simulink model "ROS2ValetControllerExample"  (R2022b)
settings: Solver=FixedStepAuto  StartTime=0.0  StopTime=inf  RelTol=1e-3
model workspace (MAT data in the model file):
  SL_ROS_VariableLengthArrays_MaxSizes.CommonInfo.ArrayTruncateAction = 'EmitWarning'
  SL_ROS_VariableLengthArrays_MaxSizes.MsgTypeMap = containers.Map
  SL_ROS_VariableLengthArrays_MaxSizes.MsgTypeMap.serialization.keys = {'std_msgs/Float64MultiArray'}
  SL_ROS_VariableLengthArrays_MaxSizes.MsgTypeMap.serialization.values{1}.PropertyName = 'data'
  SL_ROS_VariableLengthArrays_MaxSizes.MsgTypeMap.serialization.values{1}.DataType = 'double'
  SL_ROS_VariableLengthArrays_MaxSizes.MsgTypeMap.serialization.values{1}.MaxLength = 1500
  SL_ROS_VariableLengthArrays_MaxSizes.MsgTypeMap.serialization.uniformity = 0
  SL_ROS_VariableLengthArrays_MaxSizes.MsgTypeMap.serialization.keyType = 'char'
  SL_ROS_VariableLengthArrays_MaxSizes.MsgTypeMap.serialization.valueType = 'any'
values from neighbouring files (symbols this model uses):
  directions = obj.DirectionsInternal    [ExampleHelperROSValetPathAnalyzer.m]
libraries: ros2lib x19, drivingvehiclecontroller x2
settings Model: PacingRate=1000  Creator=The MathWorks, Inc.  LastModifiedBy=The MathWorks, Inc.
settings SolverCC: AlgebraicLoopSolver=TrustRegion
settings OptimizationCC: EnhancedBackFolding=on  PassReuseOutputArgsAs=Individual arguments  ZeroExternalMemoryAtStartup=off  ZeroInternalMemoryAtStartup=off  MaxStackSize=64  OptimizeBlockOrder=speed  DifferentSizesBufferReuse=on  OptimizationCustomize=off  EfficientTunableParamExpr=on
settings DebuggingCC: ParameterTunabilityLossMsg=error  UnconnectedInputMsg=warning  UnconnectedOutputMsg=warning  UnconnectedLineMsg=warning  SFMachineParentedDataDiag=warning
settings ModelReferenceCC: EnableRefExpFcnMdlSchedulingChecks=on
settings SFSimCC: SimTargetLang=C++
settings RTWCC: Description=Embedded Coder  SystemTargetFile=ert.tlc  HardwareBoard=Robot Operating System 2 (ROS 2)  TLCOptions=-aInlineSetEventsForThisBaseRateFcn=TLC_FALSE -aSuppressMultiTaskScheduler=TLC_FALSE -aRateBasedStepFcn=1  TemplateMakefile=ert_default_tmf  GenerateReport=on  Toolchain=Colcon Tools  IncludeHyperlinkInReport=on  LaunchReport=on  TargetLang=C++  GenerateTraceInfo=on  GenerateTraceReport=on  GenerateTraceReportSl=on  GenerateTraceReportSf=on  GenerateTraceReportEml=on
settings CodeAppCC: ForceParamTrailComments=on  IgnoreCustomStorageClasses=off  OperatorAnnotations=on  SimulinkDataObjDesc=on  SFDataObjDesc=on  InsertBlockDesc=on
settings ERTTargetCC: CodeInterfacePackaging=C++ class  RootIOFormat=Structure reference

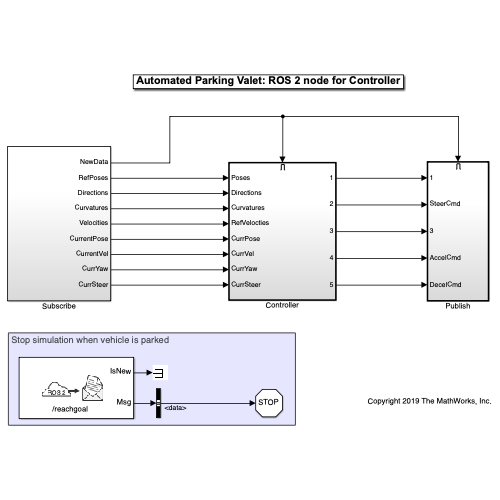
[thumbnail: Simulink's stored preview of the top-level diagram]
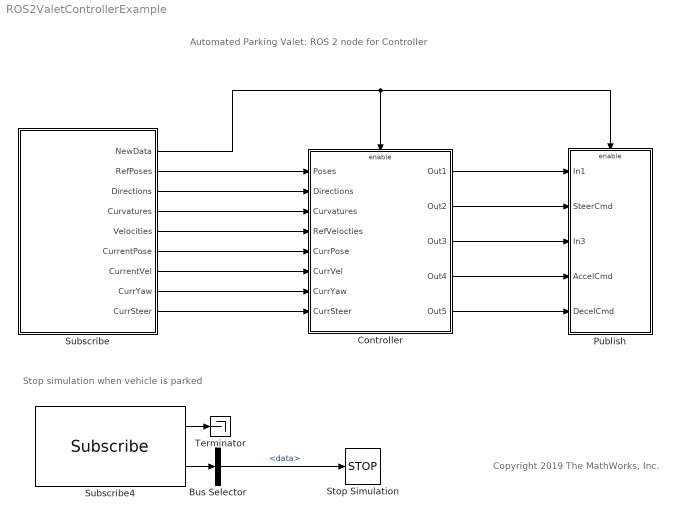
== system ROS2ValetControllerExample ==
  note: Copyright 2019 The MathWorks, Inc.
  note: Automated Parking Valet: ROS 2 node for Controller
  note: Stop simulation when vehicle is parked
  Bus Selector : BusSelector  OutputSignals=data
  Controller : Subsystem
  Publish : Subsystem
  Stop Simulation : Stop
  Subscribe : Subsystem
  Subscribe4 : ros2lib/Subscribe  topicSource=Specify your own  topic=/reachgoal  messageType=std_msgs/Bool  sampleTime=-1  QOSHistory=Keep last  QOSDepth=1  QOSReliability=Reliable  QOSDurability=Volatile
  Terminator : Terminator
  wires:
  Subscribe/1(NewData) -> Controller/Enable, Publish/Enable
  Subscribe/2(RefPoses) -> Controller/1(Poses)
  Subscribe/3(Directions) -> Controller/2(Directions)
  Subscribe/4(Curvatures) -> Controller/3(Curvatures)
  Subscribe/5(Velocities) -> Controller/4(RefVelocties)
  Subscribe/6(CurrentPose) -> Controller/5(CurrPose)
  Subscribe/7(CurrentVel) -> Controller/6(CurrVel)
  Subscribe/8(CurrYaw) -> Controller/7(CurrYaw)
  Subscribe/9(CurrSteer) -> Controller/8(CurrSteer)
  Subscribe4/2 -> Bus Selector/1
  Subscribe4/1 -> Terminator/1
  Bus Selector/1 -> Stop Simulation/1  "<data>"
  Controller/4(Out4) -> Publish/4(AccelCmd)
  Controller/5(Out5) -> Publish/5(DecelCmd)
  Controller/3(Out3) -> Publish/3(In3)
  Controller/2(Out2) -> Publish/2(SteerCmd)
  Controller/1(Out1) -> Publish/1(In1)

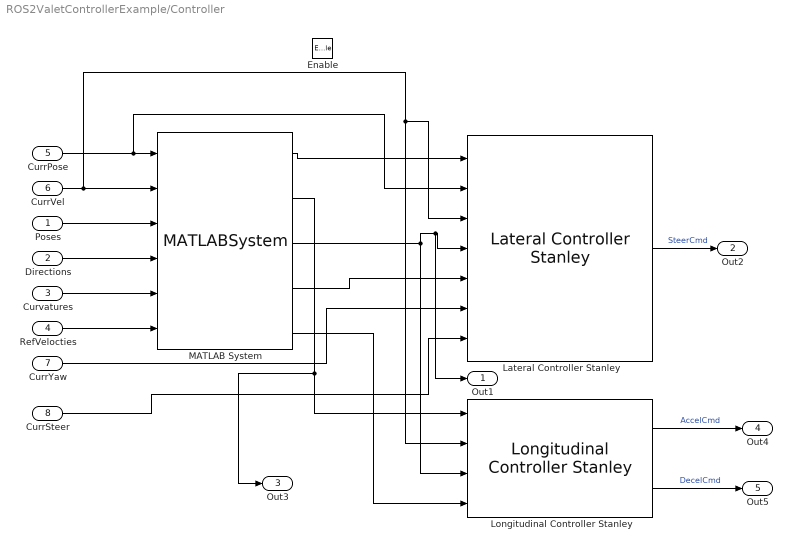
== system ROS2ValetControllerExample/Controller ==
  Poses : Inport
  Directions : Inport  Port=2
  Curvatures : Inport  Port=3
  RefVelocties : Inport  Port=4
  CurrPose : Inport  Port=5
  CurrVel : Inport  Port=6
  CurrYaw : Inport  Port=7
  CurrSteer : Inport  Port=8
  Enable : EnablePort
  Lateral Controller Stanley : drivingvehiclecontroller/Lateral Controller Stanley  ModelType=Dynamic bicycle model  PositionGainF=2  PositionGainR=2.5  YawRateGain=0.25  DelayGain=0.2  VehicleMass=1575  Lf=1.2  Lr=1.6  TireStiffness=19e3  Wheelbase=2.8  MaxSteeringAngle=35
  Longitudinal Controller Stanley : drivingvehiclecontroller/Longitudinal Controller Stanley  Kp=2.5  Ki=1  SampleTime=0.05  MaxAcceleration=3  MaxDeceleration=6
  MATLAB System : MATLABSystem  System=ExampleHelperROSValetPathAnalyzer  Wheelbase=2.8  HasResetOutput=on  SimulateUsing=Interpreted execution
      mask Type: ExampleHelperROSValetPathAnalyzer
      mask Display:
      | disp(['Helper' char(10) 'Path' char(10) 'Analyzer']);
      | port_label('input',1,'CurrPose');
      | port_label('input',2,'CurrVelocity');
      | port_label('input',3,'RefPoses');
      | port_label('input',4,'Directions');
      | port_label('input',5,'Curvatures');
      | port_label('input',6,'RefVelocities');
      | port_label('output',1,'RefPose');
      | port_label('output',2,'RefVelocity');
      | port_label('output',3,'Direction');
      | port_label('output',4,'Curvature');
      | port_label('output',5,'Reset');
  Out1 : Outport
  Out2 : Outport  Port=2
  Out3 : Outport  Port=3
  Out4 : Outport  Port=4
  Out5 : Outport  Port=5
  wires:
  MATLAB System/2 -> Longitudinal Controller Stanley/1, Out3/1
  MATLAB System/4 -> Lateral Controller Stanley/5
  MATLAB System/1 -> Lateral Controller Stanley/1
  MATLAB System/5 -> Longitudinal Controller Stanley/4
  Poses/1 -> MATLAB System/3
  CurrVel/1 -> Lateral Controller Stanley/3, Longitudinal Controller Stanley/2, MATLAB System/2
  CurrYaw/1 -> Lateral Controller Stanley/6
  CurrSteer/1 -> Lateral Controller Stanley/7
  CurrPose/1 -> Lateral Controller Stanley/2, MATLAB System/1
  Directions/1 -> MATLAB System/4
  Curvatures/1 -> MATLAB System/5
  RefVelocties/1 -> MATLAB System/6
  MATLAB System/3 -> Out1/1, Lateral Controller Stanley/4, Longitudinal Controller Stanley/3
  Lateral Controller Stanley/1 -> Out2/1  "SteerCmd"
  Longitudinal Controller Stanley/1 -> Out4/1  "AccelCmd"
  Longitudinal Controller Stanley/2 -> Out5/1  "DecelCmd"

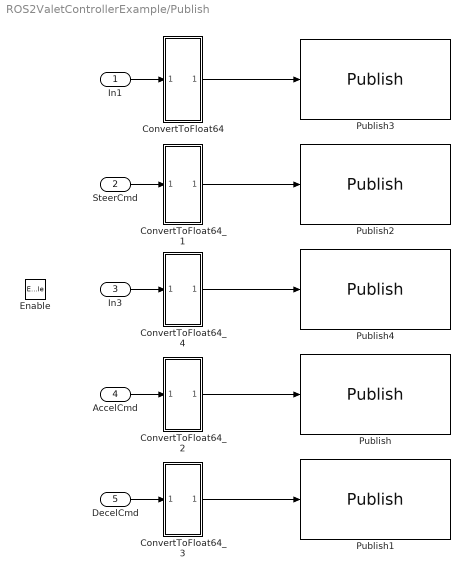
== system ROS2ValetControllerExample/Publish ==
  In1 : Inport
  SteerCmd : Inport  Port=2
  In3 : Inport  Port=3
  AccelCmd : Inport  Port=4
  DecelCmd : Inport  Port=5
  Enable : EnablePort
  ConvertToFloat64 : Subsystem
  ConvertToFloat64_1 : Subsystem
  ConvertToFloat64_2 : Subsystem
  ConvertToFloat64_3 : Subsystem
  ConvertToFloat64_4 : Subsystem
  Publish : ros2lib/Publish  topicSource=Specify your own  topic=/accelcmd  messageType=std_msgs/Float64  QOSHistory=Keep last  QOSDepth=1  QOSReliability=Reliable  QOSDurability=Volatile
  Publish1 : ros2lib/Publish  topicSource=Specify your own  topic=/decelcmd  messageType=std_msgs/Float64  QOSHistory=Keep last  QOSDepth=1  QOSReliability=Reliable  QOSDurability=Volatile
  Publish2 : ros2lib/Publish  topicSource=Specify your own  topic=/steeringangle  messageType=std_msgs/Float64  QOSHistory=Keep last  QOSDepth=1  QOSReliability=Reliable  QOSDurability=Volatile
  Publish3 : ros2lib/Publish  topicSource=Specify your own  topic=/vehdir  messageType=std_msgs/Float64  QOSHistory=Keep last  QOSDepth=1  QOSReliability=Reliable  QOSDurability=Volatile
  Publish4 : ros2lib/Publish  topicSource=Specify your own  topic=/refvelocity  messageType=std_msgs/Float64  QOSHistory=Keep last  QOSDepth=1  QOSReliability=Reliable  QOSDurability=Volatile
  wires:
  AccelCmd/1 -> ConvertToFloat64_2/1(In1)
  SteerCmd/1 -> ConvertToFloat64_1/1(In1)
  DecelCmd/1 -> ConvertToFloat64_3/1(In1)
  ConvertToFloat64_2/1(Out1) -> Publish/1
  ConvertToFloat64_4/1(Out1) -> Publish4/1
  ConvertToFloat64_1/1(Out1) -> Publish2/1
  ConvertToFloat64/1(Out1) -> Publish3/1
  In3/1 -> ConvertToFloat64_4/1(In1)
  ConvertToFloat64_3/1(Out1) -> Publish1/1
  In1/1 -> ConvertToFloat64/1(In1)

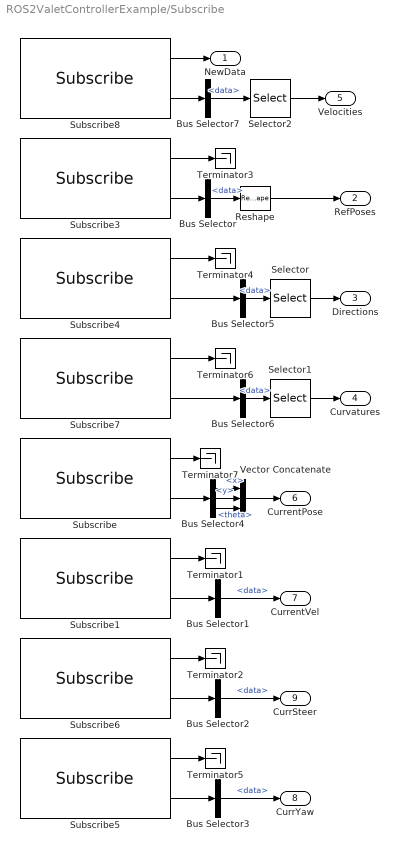
== system ROS2ValetControllerExample/Subscribe ==
  Bus Selector{,1..3,5..7} (7 alike) : BusSelector  OutputSignals=data
  Bus Selector4 : BusSelector  OutputSignals=x,y,theta
  Reshape : Reshape  OutputDimensionality=Customize  OutputDimensions=[500,3]
  Selector : Selector  InputPortWidth=1500  IndexOptions=Starting index (dialog)  Indices=1  OutputSizes=500
  Selector1 : Selector  InputPortWidth=1500  IndexOptions=Starting index (dialog)  Indices=1  OutputSizes=500
  Selector2 : Selector  InputPortWidth=1500  IndexOptions=Starting index (dialog)  Indices=1  OutputSizes=500
  Subscribe : ros2lib/Subscribe  topicSource=Select from ROS network  topic=/currentpose  messageType=geometry_msgs/Pose2D  sampleTime=-1  QOSHistory=Keep last  QOSDepth=1  QOSReliability=Reliable  QOSDurability=Volatile
  Subscribe1 : ros2lib/Subscribe  topicSource=Select from ROS network  topic=/currentvel  messageType=std_msgs/Float64  sampleTime=-1  QOSHistory=Keep last  QOSDepth=1  QOSReliability=Reliable  QOSDurability=Volatile
  Subscribe3 : ros2lib/Subscribe  topicSource=Specify your own  topic=/smoothpath  messageType=std_msgs/Float64MultiArray  sampleTime=-1  QOSHistory=Keep last  QOSDepth=1  QOSReliability=Reliable  QOSDurability=Volatile
  Subscribe4 : ros2lib/Subscribe  topicSource=Specify your own  topic=/directions  messageType=std_msgs/Float64MultiArray  sampleTime=-1  QOSHistory=Keep last  QOSDepth=1  QOSReliability=Reliable  QOSDurability=Volatile
  Subscribe5 : ros2lib/Subscribe  topicSource=Specify your own  topic=/curryawrate  messageType=std_msgs/Float64  sampleTime=-1  QOSHistory=Keep last  QOSDepth=1  QOSReliability=Reliable  QOSDurability=Volatile
  Subscribe6 : ros2lib/Subscribe  topicSource=Specify your own  topic=/currentsteering  messageType=std_msgs/Float64  sampleTime=-1  QOSHistory=Keep last  QOSDepth=1  QOSReliability=Reliable  QOSDurability=Volatile
  Subscribe7 : ros2lib/Subscribe  topicSource=Specify your own  topic=/curvatures  messageType=std_msgs/Float64MultiArray  sampleTime=-1  QOSHistory=Keep last  QOSDepth=1  QOSReliability=Reliable  QOSDurability=Volatile
  Subscribe8 : ros2lib/Subscribe  topicSource=Specify your own  topic=/velprofile  messageType=std_msgs/Float64MultiArray  sampleTime=-1  QOSHistory=Keep last  QOSDepth=1  QOSReliability=Reliable  QOSDurability=Volatile
  Terminator{1..7} (7 alike) : Terminator
  Vector Concatenate : Concatenate  NumInputs=3  Mode=Multidimensional array  ConcatenateDimension=2
  NewData : Outport  VectorParamsAs1DForOutWhenUnconnected=off
  RefPoses : Outport  Port=2  VectorParamsAs1DForOutWhenUnconnected=off
  Directions : Outport  Port=3  VectorParamsAs1DForOutWhenUnconnected=off
  Curvatures : Outport  Port=4  VectorParamsAs1DForOutWhenUnconnected=off
  Velocities : Outport  Port=5  VectorParamsAs1DForOutWhenUnconnected=off
  CurrentPose : Outport  Port=6  VectorParamsAs1DForOutWhenUnconnected=off
  CurrentVel : Outport  Port=7  VectorParamsAs1DForOutWhenUnconnected=off
  CurrYaw : Outport  Port=8  VectorParamsAs1DForOutWhenUnconnected=off
  CurrSteer : Outport  Port=9  VectorParamsAs1DForOutWhenUnconnected=off
  wires:
  Subscribe/1 -> Terminator7/1
  Subscribe1/2 -> Bus Selector1/1
  Subscribe1/1 -> Terminator1/1
  Subscribe3/1 -> Terminator3/1
  Subscribe4/1 -> Terminator4/1
  Subscribe5/1 -> Terminator5/1
  Subscribe5/2 -> Bus Selector3/1
  Subscribe6/2 -> Bus Selector2/1
  Subscribe6/1 -> Terminator2/1
  Subscribe7/1 -> Terminator6/1
  Subscribe8/1 -> NewData/1
  Bus Selector6/1 -> Selector1/1  "<data>"
  Bus Selector7/1 -> Selector2/1  "<data>"
  Bus Selector4/2 -> Vector Concatenate/2  "<y>"
  Bus Selector4/3 -> Vector Concatenate/3  "<theta>"
  Bus Selector4/1 -> Vector Concatenate/1  "<x>"
  Bus Selector5/1 -> Selector/1  "<data>"
  Subscribe/2 -> Bus Selector4/1
  Vector Concatenate/1 -> CurrentPose/1
  Bus Selector1/1 -> CurrentVel/1  "<data>"
  Bus Selector2/1 -> CurrSteer/1  "<data>"
  Bus Selector3/1 -> CurrYaw/1  "<data>"
  Bus Selector/1 -> Reshape/1  "<data>"
  Subscribe3/2 -> Bus Selector/1
  Reshape/1 -> RefPoses/1
  Subscribe4/2 -> Bus Selector5/1
  Selector/1 -> Directions/1
  Subscribe7/2 -> Bus Selector6/1
  Selector1/1 -> Curvatures/1
  Subscribe8/2 -> Bus Selector7/1
  Selector2/1 -> Velocities/1

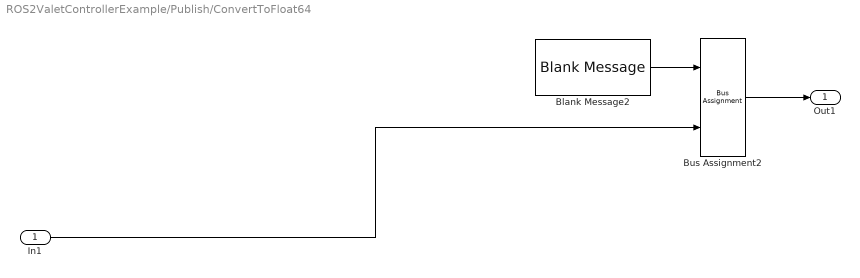
== system ROS2ValetControllerExample/Publish/ConvertToFloat64 ==
  In1 : Inport
  Blank Message2 : ros2lib/Blank Message  messageClass=Message  entityType=std_msgs/Float64  messageType=std_msgs/Float64  SampleTime=-1
  Bus Assignment2 : BusAssignment  AssignedSignals=data
  Out1 : Outport
  wires:
  Blank Message2/1 -> Bus Assignment2/1
  Bus Assignment2/1 -> Out1/1
  In1/1 -> Bus Assignment2/2

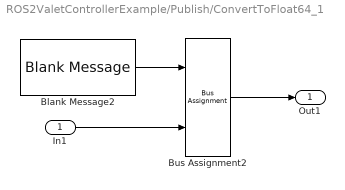
== system ROS2ValetControllerExample/Publish/ConvertToFloat64_1 ==
  In1 : Inport
  Blank Message2 : ros2lib/Blank Message  messageClass=Message  entityType=std_msgs/Float64  messageType=std_msgs/Float64  SampleTime=-1
  Bus Assignment2 : BusAssignment  AssignedSignals=data
  Out1 : Outport
  wires:
  In1/1 -> Bus Assignment2/2
  Bus Assignment2/1 -> Out1/1
  Blank Message2/1 -> Bus Assignment2/1

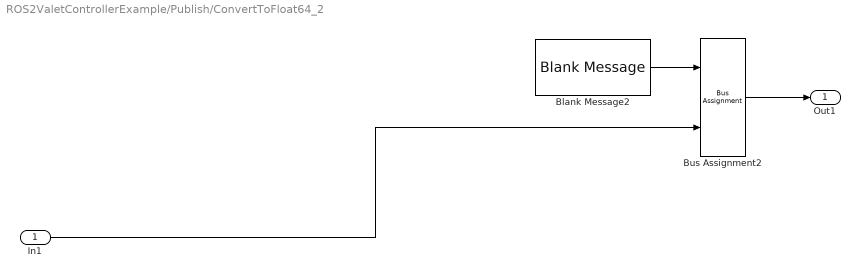
== system ROS2ValetControllerExample/Publish/ConvertToFloat64_2 ==
  In1 : Inport
  Blank Message2 : ros2lib/Blank Message  messageClass=Message  entityType=std_msgs/Float64  messageType=std_msgs/Float64  SampleTime=-1
  Bus Assignment2 : BusAssignment  AssignedSignals=data
  Out1 : Outport
  wires:
  Blank Message2/1 -> Bus Assignment2/1
  Bus Assignment2/1 -> Out1/1
  In1/1 -> Bus Assignment2/2

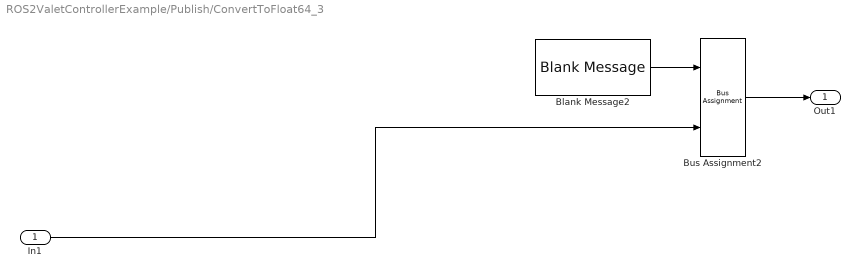
== system ROS2ValetControllerExample/Publish/ConvertToFloat64_3 ==
  In1 : Inport
  Blank Message2 : ros2lib/Blank Message  messageClass=Message  entityType=std_msgs/Float64  messageType=std_msgs/Float64  SampleTime=-1
  Bus Assignment2 : BusAssignment  AssignedSignals=data
  Out1 : Outport
  wires:
  In1/1 -> Bus Assignment2/2
  Bus Assignment2/1 -> Out1/1
  Blank Message2/1 -> Bus Assignment2/1

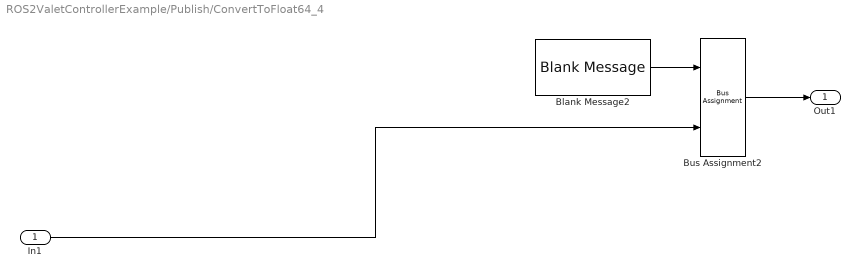
== system ROS2ValetControllerExample/Publish/ConvertToFloat64_4 ==
  In1 : Inport
  Blank Message2 : ros2lib/Blank Message  messageClass=Message  entityType=std_msgs/Float64  messageType=std_msgs/Float64  SampleTime=-1
  Bus Assignment2 : BusAssignment  AssignedSignals=data
  Out1 : Outport
  wires:
  Blank Message2/1 -> Bus Assignment2/1
  Bus Assignment2/1 -> Out1/1
  In1/1 -> Bus Assignment2/2
